simulink model "quadrotor_model_2"  (R2024b)
settings: Solver=VariableStepAuto  StartTime=0.0  StopTime=10.0  RelTol=1e-3
values from neighbouring files (symbols this model uses):
  b = 0.001    [exercise_2_simulink.m]    (also in exercise_2_simulink_2.m)
  D = diag([.01 .01 .01])    [exercise_2_simulink.m]    (also in exercise_2_simulink_2.m)
  g_i = [0 0 -9.81]'    [exercise_2_simulink.m]    (also in exercise_2_simulink_2.m)
  Ixx = 3e-6    (= 3e-06)    [exercise_2_simulink.m]    (also in exercise_2_simulink_2.m)
  Iyy = 3e-6    (= 3e-06)    [exercise_2_simulink.m]    (also in exercise_2_simulink_2.m)
  Izz = 1e-5    (= 1e-05)    [exercise_2_simulink.m]    (also in exercise_2_simulink_2.m)
  k = 0.01    [exercise_2_simulink.m]    (also in exercise_2_simulink_2.m; uas_parameters.m = 0.0176714586764)
  L = 0.225    [exercise_2_simulink.m]    (also in exercise_2_simulink_2.m)
  m = 0.5    [exercise_2_simulink.m]    (also in exercise_2_simulink_2.m)
  omega = cases{i,2}    [exercise_2_simulink.m]    (also in exercise_2_simulink_2.m)
  p0 = [0 0 0]'    [exercise_2_simulink.m]    (also in exercise_2_simulink_2.m)
  q0 = [1 0 0 0]'    [exercise_2_simulink_2.m]
  v0 = [0 0 0]'    [exercise_2_simulink.m]    (also in exercise_2_simulink_2.m)
  w0 = [0 0 0]'    [exercise_2_simulink.m]    (also in exercise_2_simulink_2.m)
settings Model: Creator=claes  LastModifiedBy=jonas

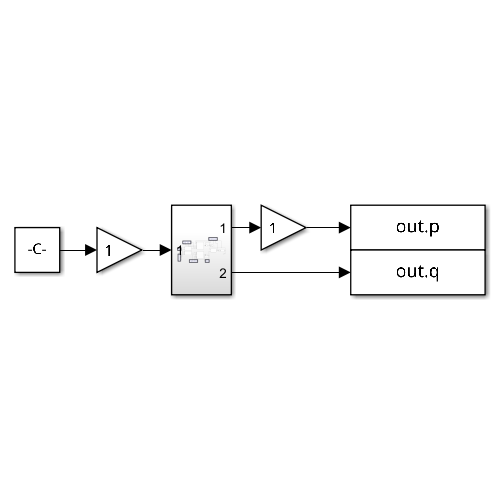
[thumbnail: Simulink's stored preview of the top-level diagram]
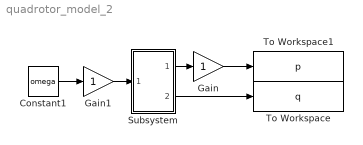
== system quadrotor_model_2 ==
  Constant1 : Constant  Value=omega
  Gain : Gain
  Gain1 : Gain
  Subsystem : Subsystem
  To Workspace : ToWorkspace  VariableName=q  SaveFormat=Timeseries  SampleTime=-1
  To Workspace1 : ToWorkspace  VariableName=p  SaveFormat=Timeseries  SampleTime=-1
  wires:
  Constant1/1 -> Gain1/1
  Subsystem/2(Out2) -> To Workspace/1
  Gain/1 -> To Workspace1/1
  Subsystem/1(Out1) -> Gain/1
  Gain1/1 -> Subsystem/1(In1)

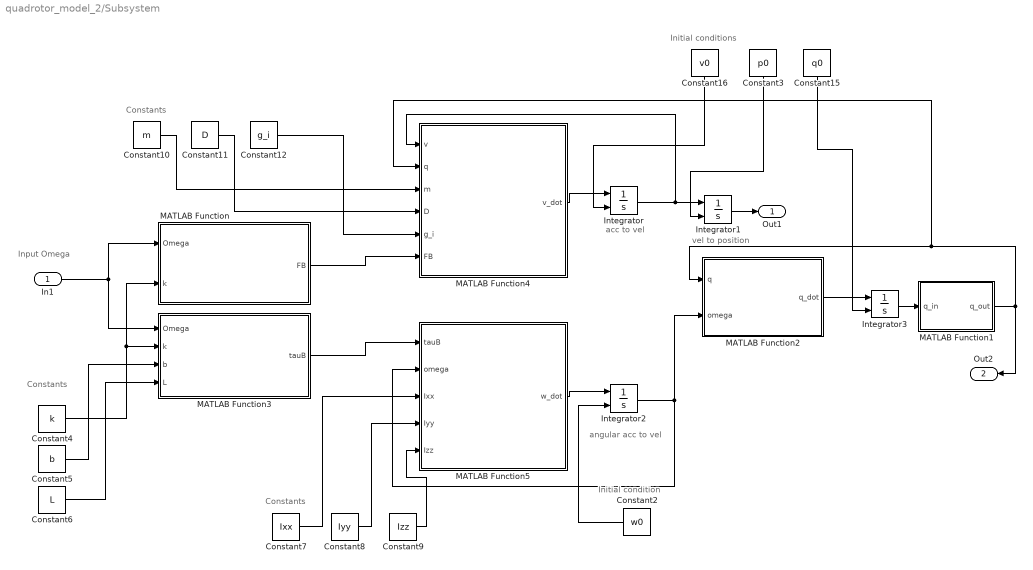
== system quadrotor_model_2/Subsystem ==
  note: angular acc to vel
  note: Initial condition
  note: Input Omega
  note: Constants
  note: Constants
  note: Constants
  note: Initial conditions
  note: acc to vel
  note: vel to position
  In1 : Inport
  Constant10 : Constant  Value=m
  Constant11 : Constant  Value=D
  Constant12 : Constant  Value=g_i
  Constant15 : Constant  Value=q0
  Constant16 : Constant  Value=v0
  Constant2 : Constant  Value=w0
  Constant3 : Constant  Value=p0
  Constant4 : Constant  Value=k
  Constant5 : Constant  Value=b
  Constant6 : Constant  Value=L
  Constant7 : Constant  Value=Ixx
  Constant8 : Constant  Value=Iyy
  Constant9 : Constant  Value=Izz
  Integrator : Integrator  InitialConditionSource=external
  Integrator1 : Integrator  InitialConditionSource=external
  Integrator2 : Integrator  InitialConditionSource=external  InitialCondition=w0
  Integrator3 : Integrator  InitialConditionSource=external
  MATLAB Function : MATLAB Function  TreatAsAtomicUnit=on
  MATLAB Function1 : MATLAB Function  TreatAsAtomicUnit=on
  MATLAB Function2 : MATLAB Function  TreatAsAtomicUnit=on
  MATLAB Function3 : MATLAB Function  TreatAsAtomicUnit=on
  MATLAB Function4 : MATLAB Function  TreatAsAtomicUnit=on
  MATLAB Function5 : MATLAB Function  TreatAsAtomicUnit=on
  Out1 : Outport
  Out2 : Outport  Port=2
  wires:
  MATLAB Function2/1(q_dot) -> Integrator3/1
  Constant5/1 -> MATLAB Function3/3(b)
  Integrator/1 -> MATLAB Function4/1(v), Integrator1/1
  MATLAB Function5/1(w_dot) -> Integrator2/1
  In1/1 -> MATLAB Function3/1(Omega), MATLAB Function/1(Omega)
  Integrator2/1 -> MATLAB Function2/2(omega), MATLAB Function5/2(omega)
  Constant6/1 -> MATLAB Function3/4(L)
  Integrator1/1 -> Out1/1
  Constant16/1 -> Integrator/2
  Constant15/1 -> Integrator3/2
  MATLAB Function1/1(q_out) -> Out2/1, MATLAB Function2/1(q), MATLAB Function4/2(q)
  Constant2/1 -> Integrator2/2
  Constant10/1 -> MATLAB Function4/3(m)
  Constant9/1 -> MATLAB Function5/5(Izz)
  Constant8/1 -> MATLAB Function5/4(Iyy)
  Constant7/1 -> MATLAB Function5/3(Ixx)
  MATLAB Function3/1(tauB) -> MATLAB Function5/1(tauB)
  Constant4/1 -> MATLAB Function/2(k), MATLAB Function3/2(k)
  MATLAB Function/1(FB) -> MATLAB Function4/6(FB)
  Integrator3/1 -> MATLAB Function1/1(q_in)
  Constant11/1 -> MATLAB Function4/4(D)
  Constant12/1 -> MATLAB Function4/5(g_i)
  MATLAB Function4/1(v_dot) -> Integrator/1
  Constant3/1 -> Integrator1/2

== matlab function quadrotor_model_2/Subsystem/MATLAB Function1 ==
  data: q_in input; q_out output
% MATLAB-Function   q_norm
function q_out = q_norm(q_in)
n = norm(q_in);
if n==0, n = 1; end      % safety
q_out = q_in./n;

== matlab function quadrotor_model_2/Subsystem/MATLAB Function ==
  data: Omega input; FB output; k input
function FB  = forces(Omega, k)
    % omega = [ω1 ω2 ω3 ω4]'  (rad/s)
    T = k*sum(Omega.^2);      % total thrust magnitude
    FB = [0;0;T];             % thrust in body frame (z_b)
end

== matlab function quadrotor_model_2/Subsystem/MATLAB Function2 ==
  data: q input; q_dot output; omega input
function q_dot = q_kin(q, omega)
% q      : 4×1  [η; εx; εy; εz]  (unit quaternion, scalar-first)
% omega  : 3×1  body angular velocity [rad/s]
% q_dot  : 4×1

eta = q(1);  ex = q(2);  ey = q(3);  ez = q(4);
wx  = omega(1); wy = omega(2); wz = omega(3);

q_dot = 0.5 * [ -ex*wx - ey*wy - ez*wz;
                 eta*wx + ey*wz - ez*wy;
                 eta*wy + ez*wx - ex*wz;
                 eta*wz + ex*wy - ey*wx ];
end

== matlab function quadrotor_model_2/Subsystem/MATLAB Function3 ==
  data: Omega input; tauB output; k input; b input; L input
function tauB  = torques(Omega, k, b, L)
    % omega = [ω1 ω2 ω3 ω4]'  (rad/s)
    tauB = [ L*k*(Omega(1)^2 - Omega(3)^2);     % roll
             L*k*(Omega(2)^2 - Omega(4)^2);     % pitch
             b*(Omega(1)^2 - Omega(2)^2 + Omega(3)^2 - Omega(4)^2) ];
end

== matlab function quadrotor_model_2/Subsystem/MATLAB Function4 ==
  data: v input; q input; m input; D input; g_i input; FB input; v_dot output
function v_dot = transl_dynamics(v, q, m, D, g_i, FB)
% FB      : 3×1    (N)   thrust expressed in the BODY frame
% v       : 3×1    (m/s) inertial linear velocity
% eul_a   : 3x1 (rad)   Euler angles [phi; theta; psi] representing
%                             the orientation of the body-fixed frame w.r.t.
%                             the inertial frame.
%                             phi   : roll angle
%                             theta : pitch angle
%                             psi   : yaw angle
% m       : mass
% D       : 3×3 drag matrix
% g_i     : 3×1 gravity in inertial frame

[eta, ex, ey, ez] = deal(q(1), q(2), q(3), q(4));

R = [ eta^2+ex^2-ey^2-ez^2 , 2*(ex*ey-eta*ez) , 2*(ex*ez+eta*ey);
      2*(ex*ey+eta*ez)     , eta^2-ex^2+ey^2-ez^2 , 2*(ey*ez-eta*ex);
      2*(ex*ez-eta*ey)     , 2*(ey*ez+eta*ex)     , eta^2-ex^2-ey^2+ez^2 ];
FB_i = R * FB;

% 2) drag (already in inertial frame)
FD_i = -D * v;

% 3) Newton
v_dot = (1/m)*( FB_i + FD_i ) + g_i;
end

== matlab function quadrotor_model_2/Subsystem/MATLAB Function5 ==
  data: tauB input; omega input; w_dot output; Ixx input; Iyy input; Izz input
function w_dot = rot_dynamics(tauB, omega, Ixx, Iyy, Izz)
% tauB : 3×1   (N·m)      body torques
% omega: 3×1   (rad/s)    current body angular velocity

I  = diag([Ixx Iyy Izz]);
invI = diag([1/Ixx 1/Iyy 1/Izz]);

w_cross_Iw = [  0       -omega(3)  omega(2);
                omega(3)  0       -omega(1);
               -omega(2)  omega(1) 0 ] * (I*omega);

w_dot = invI * ( tauB - w_cross_Iw );
end
